simulink model "fermentation"  (R2019b)
settings: Solver=FixedStepAuto  StartTime=0.0  StopTime=stopTime  FixedStep=timeDelta  RelTol=1e-3
values from neighbouring files (symbols this model uses):
  a = 1000    [LoadDefaults.m]
  alpha0 = 70    [LoadDefaults.m]
  alpha1 = 0.143    [LoadDefaults.m]
  alpha2 = 4e-7    (= 4e-07)    [LoadDefaults.m]
  alpha3 = 1e-4    (= 0.0001)    [LoadDefaults.m]
  b = 0.6    [LoadDefaults.m]
  beta0 = 0.4    [LoadDefaults.m]
  Cab = Ca    (= 3)    [LoadDefaults.m]
  CL_init = GenRandomWithinRange ( CL_optimal)    [GenerateHistoricalBatches.m]    (also in LoadDefaults.m = 1.16)
  CLsat = 1.16    [LoadDefaults.m]
  CO2_init = 0.5    [LoadDefaults.m]
  Ed = 50000    [LoadDefaults.m]
  Eg = 5100    [LoadDefaults.m]
  F_init = 0    [LoadDefaults.m]
  Fa_init = 0    [LoadDefaults.m]
  Fa_max = 0.01/1000    (= 1e-05)    [LoadDefaults.m]
  Fb_init = 0    [LoadDefaults.m]
  Fb_max = 100/1000    (= 0.1)    [LoadDefaults.m]
  Fc_init = 0    [LoadDefaults.m]
  gamma0 = 1e-5    (= 1e-05)    [LoadDefaults.m]
  H_init = 10^(-pH_init)    [GenerateHistoricalBatches.m]    (also in LoadDefaults.m = 1e-05)
  K = 0.04    [LoadDefaults.m]
  K1 = 1e-10    [LoadDefaults.m]
  K2 = 7e-5    (= 7e-05)    [LoadDefaults.m]
  Kc_acid = 1e-4    (= 0.0001)    [LoadDefaults.m]
  Kc_base = 8e-4    (= 0.0008)    [LoadDefaults.m]
  Kc_cooling = 7    [LoadDefaults.m]
  kd = 1e33    (= 1e+33)    [LoadDefaults.m]
  kg = 7e3    (= 7000)    [LoadDefaults.m]
  KI = 0.1    [LoadDefaults.m]
  Kop = Kop_lim    (= 0.0005)    [LoadDefaults.m]
  Kox = Kox_lim    (= 0.02)    [LoadDefaults.m]
  Kp = 0.0002    [LoadDefaults.m]
  Kx = 0.15    [LoadDefaults.m]
  lambda0 = 1.0039e-4    (= 0.00010039)    [LoadDefaults.m]
  mo = 0.467    [LoadDefaults.m]
  mu_p = 0.005    [LoadDefaults.m]
  mu_x = 0.092    [LoadDefaults.m]
  mx = 0.014    [LoadDefaults.m]
  p = 3    [LoadDefaults.m]
  P_init = 0    [LoadDefaults.m]
  P_threshold = 1.3    [LoadDefaults.m]
  pH_init = GenRandomWithinRange ( pH_optimal )    [GenerateHistoricalBatches.m]    (also in LoadDefaults.m = -log10(H_init))
  q = 0    [LoadDefaults.m]
  Qrxn_init = 0    [LoadDefaults.m]
  R = 1.987    [LoadDefaults.m]
  rhoCp = 1500    [LoadDefaults.m]
  rq2 = 1.6783e-4    (= 0.00016783)    [LoadDefaults.m]
  S_init = GenRandomWithinRange ( S_optimal )    [GenerateHistoricalBatches.m]
  S_threshold = GenRandomWithinRange ( S_threshold_range )    [GenerateHistoricalBatches.m]    (also in LoadDefaults.m = 0.3)
  setpoint_H = 10^(-1*setpoint_pH)    (= 1e-05)    [LoadDefaults.m]
  setpoint_pH = 5    [LoadDefaults.m]
  setpoint_temp = 298    [LoadDefaults.m]
  setpointGap_pH = 0.01    [LoadDefaults.m]
  sf = 600    [LoadDefaults.m]
  T0 = 273    [LoadDefaults.m]
  T_init = 298    [LoadDefaults.m]
  tauD_acid = 0.125    [LoadDefaults.m]
  tauD_base = 0.2625    [LoadDefaults.m]
  tauD_cooling = 1.6    [LoadDefaults.m]
  tauI_acid = 8.4    [LoadDefaults.m]
  tauI_base = 4.2    [LoadDefaults.m]
  tauI_cooling = 0.5    [LoadDefaults.m]
  Tc = 273+16.8    (= 289.8)    [LoadDefaults.m]
  Th = 273+50    (= 323)    [LoadDefaults.m]
  timeDelta = 0.01    [LoadDefaults.m]
  Tv = 373    [LoadDefaults.m]
  V_init = GenRandomWithinRange ( V_optimal )    [GenerateHistoricalBatches.m]    (also in LoadDefaults.m = 100)
  X_init = GenRandomWithinRange ( X_range )    [GenerateHistoricalBatches.m]    (also in LoadDefaults.m = 0.1)
  Ypo = 0.20    (= 0.2)    [LoadDefaults.m]
  Yps = 0.90    (= 0.9)    [LoadDefaults.m]
  Yxo = 0.04    [LoadDefaults.m]
  Yxs = 0.45    [LoadDefaults.m]
undefined symbols (not defined in the file or in its folder): G_O2_mean, G_O2_std, rho_cCp_c, rq1
settings Model: Creator=Jedd  LastModifiedBy=jorsmond
settings DebuggingCC: SignalInfNanChecking=error

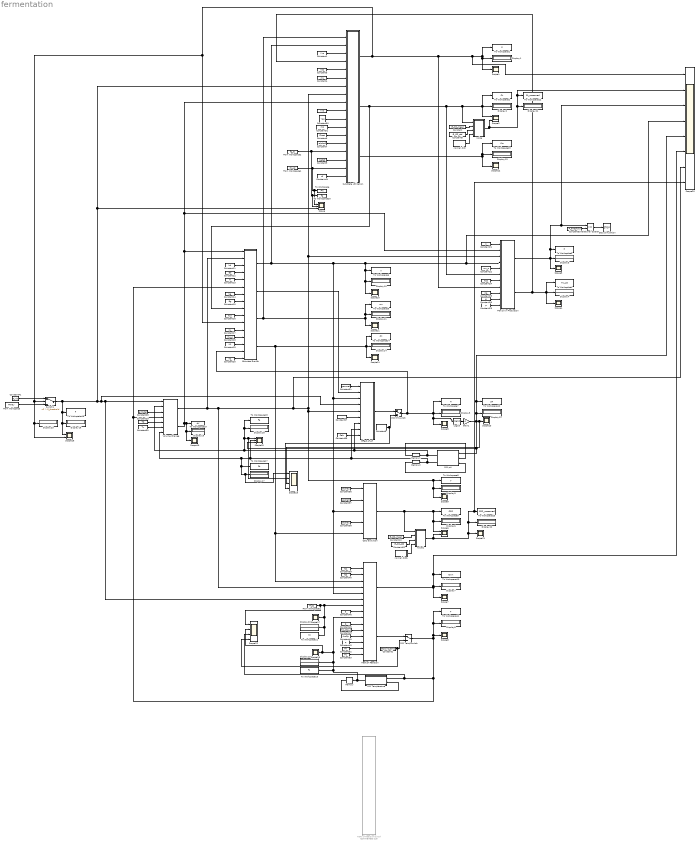
== system fermentation ==
  " " : Constant  Value=Yxo
  Biomass Growth : Subsystem
  CO2 evolution : Subsystem
  Constant : Constant  Value=G_O2_mean
  Constant1 : Constant  Value=Yxs
  Constant10 : Constant  Value=G_O2_mean
  Constant11 : Constant  Value=kd
  Constant12 : Constant  Value=Ed
  Constant13 : Constant  Value=R
  Constant14 : Constant  Value=kg
  Constant15 : Constant  Value=Eg
  Constant16 : Constant  Value=Kox
  Constant17 : Constant  Value=Kx
  Constant18 : Constant  Value=mu_x
  Constant19 : Constant  Value=K1
  Constant2 : Constant  Value=setpoint_temp
  Constant20 : Constant  Value=K2
  Constant21 : Constant  Value=K
  Constant22 : Constant  Value=mu_p
  Constant23 : Constant  Value=p
  Constant24 : Constant  Value=Kop
  Constant25 : Constant  Value=Kp
  Constant26 : Constant  Value=KI
  Constant27 : Constant  Value=timeDelta
  Constant28 : Constant  Value=lambda0
  Constant29 : Constant  Value=T0
  Constant3 : Constant  Value=Yps
  Constant30 : Constant  Value=Tv
  Constant31 : Constant  Value=gamma0
  Constant32 : Constant  Value=G_O2_std
  Constant33 : Constant  Value=P_threshold
  Constant35 : Constant  Value=Cab
  Constant36 : Constant  Value=alpha2
  Constant37 : Constant  Value=alpha3
  Constant38 : Constant  Value=alpha1
  Constant39 : Constant  Value=rq1
  Constant4 : Constant  Value=mx
  Constant40 : Constant  Value=rq2
  Constant41 : Constant  Value=F_init
  Constant43 : Constant  Value=q
  Constant44 : Constant  Value=sf
  Constant45 : Constant  Value=rhoCp
  Constant46 : Constant  Value=a
  Constant48 : Constant  Value=b
  Constant49 : Constant  Value=rho_cCp_c
  Constant5 : Constant  Value=setpoint_H
  Constant50 : Constant  Value=Ypo
  Constant51 : Constant  Value=mo
  Constant52 : Constant  Value=Th
  Constant53 : Constant  Value=Tc
  Constant6 : Constant  Value=CLsat
  Constant7 : Constant  Value=alpha0
  Constant8 : Constant  Value=G_O2_std
  Constant9 : Constant  Value=beta0
  Display{1..23} (23 alike) : Display
  Effect of pH : Subsystem
  From Workspace : FromWorkspace  VariableName=FArray  SampleTime=0
  From Workspace1 : FromWorkspace  VariableName=Pw_ts  SampleTime=timeDelta
  From Workspace2 : FromWorkspace  VariableName=fg_ts  SampleTime=timeDelta
  From Workspace3 : FromWorkspace  VariableName=Tf_ts  SampleTime=timeDelta
  Gain1 : Gain  Gain=-1
  Heat of Reaction : Subsystem
  Heat of Reaction(Cinar) : Subsystem  Commented=on
  Log10 : Math  Operator=log10  SignedPower=off  SaturateOnIntegerOverflow=on
  Memory : Memory  InitialCondition=Fc_init
  Memory1 : Memory  InitialCondition=Fa_init
  Memory2 : Memory  InitialCondition=Fb_init
  PID Temp switch : ManualSwitch
  PID Temperature : Subsystem
  PID [H] switch : ManualSwitch
  PID pH : Subsystem
  Penicillin Production : Subsystem
  Relational Operator : RelationalOperator  OutDataTypeStr=boolean  RndMeth=Simplest
  Scope : Scope  NumInputPorts=3
  Scope{1,3..5,7..15,17,19,21} (16 alike) : Scope
  Scope16 : Scope  NumInputPorts=2
  Scope18 : Scope  NumInputPorts=3
  Scope2 : Scope  NumInputPorts=2
  Scope20 : Scope  NumInputPorts=8
  Scope22 : Scope  NumInputPorts=4
  Scope23 : Scope  NumInputPorts=4
  Scope6 : Scope  NumInputPorts=2
  Stop Simulation : Stop
  Substrate Utilization : Subsystem
  Switch1 : Switch  Criteria=u2 > Threshold  Threshold=S_threshold
  To Workspace : ToWorkspace  VariableName=Pw  SaveFormat=Timeseries  SampleTime=-1
  To Workspace1 : ToWorkspace  VariableName=S  SaveFormat=Timeseries  SampleTime=-1
  To Workspace10 : ToWorkspace  VariableName=Qrxn  SaveFormat=Timeseries  SampleTime=-1
  To Workspace11 : ToWorkspace  VariableName=T  SaveFormat=Timeseries  SampleTime=-1
  To Workspace12 : ToWorkspace  VariableName=pH  SaveFormat=Timeseries  SampleTime=-1
  To Workspace13 : ToWorkspace  VariableName=Kla  SaveFormat=Timeseries  SampleTime=-1
  To Workspace14 : ToWorkspace  VariableName=dX  SaveFormat=Timeseries  SampleTime=-1
  To Workspace15 : ToWorkspace  VariableName=Fc  SaveFormat=Timeseries  SampleTime=-1
  To Workspace16 : ToWorkspace  VariableName=F  SaveFormat=Timeseries  SampleTime=-1
  To Workspace17 : ToWorkspace  VariableName=Fb  SaveFormat=Timeseries  SampleTime=-1
  To Workspace18 : ToWorkspace  VariableName=Fa  SaveFormat=Timeseries  SampleTime=-1
  To Workspace19 : ToWorkspace  VariableName=dV  SaveFormat=Timeseries  SampleTime=-1
  To Workspace2 : ToWorkspace  VariableName=CL  SaveFormat=Timeseries  SampleTime=-1
  To Workspace20 : ToWorkspace  VariableName=fg  SaveFormat=Timeseries  SampleTime=-1
  To Workspace21 : ToWorkspace  VariableName=Tf  SaveFormat=Timeseries  SampleTime=-1
  To Workspace22 : ToWorkspace  VariableName=CL_measured  SaveFormat=Timeseries  SampleTime=-1
  To Workspace23 : ToWorkspace  VariableName=CO2_measured  SaveFormat=Timeseries  SampleTime=-1
  To Workspace3 : ToWorkspace  VariableName=P  SaveFormat=Timeseries  SampleTime=-1
  To Workspace4 : ToWorkspace  VariableName=mu_pp  SaveFormat=Timeseries  SampleTime=-1
  To Workspace5 : ToWorkspace  VariableName=mu  SaveFormat=Timeseries  SampleTime=-1
  To Workspace6 : ToWorkspace  VariableName=X  SaveFormat=Timeseries  SampleTime=-1
  To Workspace7 : ToWorkspace  VariableName=H  SaveFormat=Timeseries  SampleTime=-1
  To Workspace8 : ToWorkspace  VariableName=V  SaveFormat=Timeseries  SampleTime=-1
  To Workspace9 : ToWorkspace  VariableName=CO2  SaveFormat=Timeseries  SampleTime=-1
  Volume Change : Subsystem
  noise : MATLAB Function  TreatAsAtomicUnit=on
  noise1 : MATLAB Function  TreatAsAtomicUnit=on
  normal dist : MATLAB Function  TreatAsAtomicUnit=on
  normal dist1 : MATLAB Function  TreatAsAtomicUnit=on
  wires:
  Biomass Growth/2(mu*X) -> Effect of pH/2(mu*X)
  Biomass Growth/4(dX/dt) -> Heat of Reaction/3(dX/dt), CO2 evolution/5(dX/dt), To Workspace14/1, Scope14/1, Display14/1
  Volume Change/2(dV/dt) -> Scope19/1, Display19/1, To Workspace19/1, Biomass Growth/1(dV/dt), Penicillin Production/2(dV/dt), Substrate Utilization/9(dV/dt)
  Constant1/1 -> Substrate Utilization/3(Yxs)
  Penicillin Production/2(mu_pp) -> Substrate Utilization/4(mu_pp), To Workspace4/1, Scope4/1, Display4/1
  Constant3/1 -> Substrate Utilization/5(Yps)
  Constant4/1 -> Substrate Utilization/6(mx)
  " "/1 -> Substrate Utilization/10(Yxo)
  Constant50/1 -> Substrate Utilization/11(Ypo)
  Constant51/1 -> Substrate Utilization/12(mo)
  Constant6/1 -> Substrate Utilization/13(CLsat)
  Constant7/1 -> Substrate Utilization/14(alpha0)
  From Workspace2/1 -> Scope/2, To Workspace20/1, Substrate Utilization/15(fg)
  Constant9/1 -> Substrate Utilization/16(beta0)
  From Workspace1/1 -> Scope/1, To Workspace/1, Substrate Utilization/17(Pw)
  Constant11/1 -> Biomass Growth/3(kd)
  Constant12/1 -> Biomass Growth/4(Ed)
  Constant13/1 -> Biomass Growth/5(R)
  Constant14/1 -> Biomass Growth/7(kg)
  Constant15/1 -> Biomass Growth/8(Eg)
  Constant16/1 -> Biomass Growth/10(Kox)
  Constant17/1 -> Biomass Growth/12(Kx)
  Constant18/1 -> Biomass Growth/13(mu_x)
  Constant19/1 -> Biomass Growth/14(K1)
  Constant20/1 -> Biomass Growth/16(K2)
  Constant21/1 -> Penicillin Production/1(K)
  Constant22/1 -> Penicillin Production/5(mu_p)
  Constant24/1 -> Penicillin Production/7(Kop)
  Constant25/1 -> Penicillin Production/9(Kp)
  Constant26/1 -> Penicillin Production/10(KI)
  Switch1/1 -> Scope16/1, Display16/1, To Workspace16/1, Substrate Utilization/7(F), Scope/3, Effect of pH/4(F), Heat of Reaction/6(F), Volume Change/1(F)  "F"
  Constant28/1 -> Volume Change/3(lambda0)
  Constant29/1 -> Volume Change/5(T0)
  Constant31/1 -> Effect of pH/1(gamma)
  Constant35/1 -> Effect of pH/9(Cab)
  Constant36/1 -> CO2 evolution/1(alpha2)
  Constant37/1 -> CO2 evolution/2(alpha3)
  Constant38/1 -> CO2 evolution/4(alpha1)
  Constant39/1 -> Heat of Reaction/1(rq1)
  Constant40/1 -> Heat of Reaction/2(rq2)
  From Workspace3/1 -> Scope22/1, To Workspace21/1, Display20/1, Scope17/1, Heat of Reaction/7(Tf)  "substrate feed temp"
  Constant45/1 -> Heat of Reaction/12(rhoCp)
  Constant46/1 -> Heat of Reaction/8(a)
  Constant48/1 -> Heat of Reaction/10(b)
  PID Temp switch/1 -> Biomass Growth/6(T), Volume Change/4(T), Scope22/3, PID Temperature/1(T), To Workspace11/1, Display8/1, Scope8/1  "T"
  Biomass Growth/1(X) -> Scope20/4, Penicillin Production/4(X), Scope10/1, Display10/1, To Workspace6/1, CO2 evolution/3(X), Heat of Reaction/5(X), Effect of pH/3(X), Substrate Utilization/2(X)  "biomass"
  Biomass Growth/3(mu) -> Substrate Utilization/1(mu), Scope11/1, To Workspace5/1, Display11/1
  Penicillin Production/1(P) -> Scope20/3, Relational Operator/1, To Workspace3/1, Scope3/1, Display3/1  "Penicillin"
  Constant49/1 -> Heat of Reaction/11(rho_cCp_c)
  Constant44/1 -> Substrate Utilization/18(sf)
  Heat of Reaction/2(T) -> PID Temp switch/1  "T"
  Constant2/1 -> Scope22/4, PID Temp switch/2
  Constant30/1 -> Volume Change/6(Tv)
  Effect of pH/1(H) -> PID [H] switch/1
  Constant5/1 -> Scope23/4, PID [H] switch/2  "SP"
  Constant23/1 -> Penicillin Production/11(p)
  Constant27/1 -> Effect of pH/6(timeDelta)
  Constant41/1 -> Switch1/1
  Substrate Utilization/1(S) -> Display23/1, Scope16/2, Switch1/2, Biomass Growth/11(S), Penicillin Production/8(S), Scope20/1, Scope1/1, Display1/1, To Workspace1/1  "Substrate"
  Constant43/1 -> Heat of Reaction/13(q)
  Constant52/1 -> Heat of Reaction/14(Th)
  Constant53/1 -> Heat of Reaction/15(Tc)
  PID [H] switch/1 -> Biomass Growth/15(H), Log10/1, Scope5/1, Display5/1, To Workspace7/1  "H"
  Log10/1 -> Gain1/1
  Volume Change/1(V) -> Heat of Reaction/4(V), Scope20/7, Effect of pH/5(V), Scope9/1, Display9/1, To Workspace8/1, Substrate Utilization/8(V), Penicillin Production/3(V), Biomass Growth/2(V)  "V"
  Substrate Utilization/3(Kla) -> Display13/1, To Workspace13/1, Scope12/1
  Heat of Reaction/1(Qrxn) -> Display7/1, Scope20/6, To Workspace10/1, Scope7/1  "Qrxn"
  Gain1/1 -> PID pH/1(PH), Scope18/3, Scope23/3, Scope13/1, Scope20/5, To Workspace12/1, Display12/1  "pH"
  Memory/1 -> PID Temperature/2(Fc,old)  "Fc(n-1)"
  PID Temperature/1(Fc,new) -> To Workspace15/1, Display15/1, Scope22/2, Scope15/1, Heat of Reaction/9(Fch), Memory/1  "Fc(n)"
  Memory1/1 -> PID pH/2(Fa,old)  "Fa(n-1)"
  Memory2/1 -> PID pH/3(Fb,old)  "Fb(n-1)"
  PID pH/1(Fa,new) -> To Workspace18/1, Display18/1, Scope23/2, Scope18/1, Volume Change/2(Fa), Effect of pH/7(Fa), Memory1/1  "Fa(n)"
  PID pH/2(Fb,new) -> Scope18/2, Scope23/1, Display17/1, To Workspace17/1, Volume Change/7(Fb), Effect of pH/8(Fb), Memory2/1  "Fb(n)"
  noise/1(y) -> Scope2/2, Display21/1, Scope20/2, To Workspace22/1  "Dissolved Oxygen"
  Substrate Utilization/2(CL) -> Biomass Growth/9(CL), Penicillin Production/6(CL), noise/1(u), Scope2/1, To Workspace2/1, Display2/1
  Constant/1 -> noise/2(mean)
  Constant8/1 -> noise/3(std)
  normal dist/1(y) -> noise/4(r)
  Constant32/1 -> noise1/3(std)
  Constant10/1 -> noise1/2(mean)
  normal dist1/1(y) -> noise1/4(r)
  CO2 evolution/1(CO2) -> noise1/1(u), Scope6/1, Display6/1, To Workspace9/1
  noise1/1(y) -> Scope6/2, Scope20/8, To Workspace23/1, Display22/1, Scope21/1  "CO2"
  Constant33/1 -> Relational Operator/2
  Relational Operator/1 -> Stop Simulation/1
  From Workspace/1 -> Switch1/3

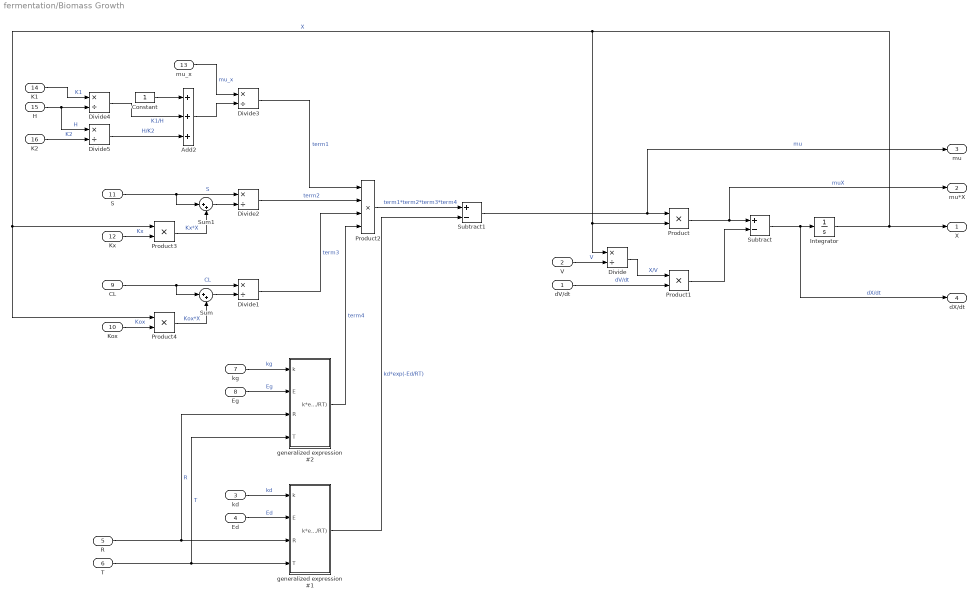
== system fermentation/Biomass Growth ==
  dV/dt : Inport
  V : Inport  Port=2
  kd : Inport  Port=3
  Ed : Inport  Port=4
  R : Inport  Port=5
  T : Inport  Port=6
  kg : Inport  Port=7
  Eg : Inport  Port=8
  CL : Inport  Port=9
  Kox : Inport  Port=10
  S : Inport  Port=11
  Kx : Inport  Port=12
  mu_x : Inport  Port=13
  K1 : Inport  Port=14
  H : Inport  Port=15
  K2 : Inport  Port=16
  Add2 : Sum  Inputs=3
  Constant : Constant
  Divide{,1..5} (6 alike) : Product  Inputs=*/
  Integrator : Integrator  InitialCondition=X_init
  Product{,1,3..4} (4 alike) : Product
  Product2 : Product  Inputs=4
  Subtract : Sum  Inputs=+-
  Subtract1 : Sum  Inputs=+-
  Sum : Sum  Inputs=|++
  Sum1 : Sum  Inputs=|++
  generalized expression #1 : Subsystem
  generalized expression #2 : Subsystem
  X : Outport
  mu*X : Outport  Port=2
  mu : Outport  Port=3
  dX/dt : Outport  Port=4
  wires:
  Product2/1 -> Subtract1/1  "term1*term2*term3*term4"
  Product/1 -> mu*X/1, Subtract/1  "muX"
  Divide/1 -> Product1/1  "X/V"
  Subtract/1 -> dX/dt/1, Integrator/1  "dX/dt"
  dV/dt/1 -> Product1/2  "dV/dt"
  V/1 -> Divide/2  "V"
  Product1/1 -> Subtract/2
  kd/1 -> generalized expression #1/1(k)  "kd"
  Ed/1 -> generalized expression #1/2(E)  "Ed"
  generalized expression #1/1(k*exp(-E/RT)) -> Subtract1/2  "kd*exp(-Ed/RT)"
  generalized expression #2/1(k*exp(-E/RT)) -> Product2/4  "term4"
  kg/1 -> generalized expression #2/1(k)  "kg"
  Eg/1 -> generalized expression #2/2(E)  "Eg"
  T/1 -> generalized expression #2/4(T), generalized expression #1/4(T)  "T"
  R/1 -> generalized expression #2/3(R), generalized expression #1/3(R)  "R"
  Subtract1/1 -> mu/1, Product/1  "mu"
  Divide1/1 -> Product2/3  "term3"
  CL/1 -> Sum/1, Divide1/1  "CL"
  Sum/1 -> Divide1/2
  Product4/1 -> Sum/2  "Kox*X"
  Kox/1 -> Product4/2  "Kox"
  Integrator/1 -> Divide/1, Product/2, Product4/1, Product3/1, X/1  "X"
  Kx/1 -> Product3/2  "Kx"
  Product3/1 -> Sum1/2  "Kx*X"
  Sum1/1 -> Divide2/2
  S/1 -> Sum1/1, Divide2/1  "S"
  Divide2/1 -> Product2/2  "term2"
  Divide3/1 -> Product2/1  "term1"
  mu_x/1 -> Divide3/1  "mu_x"
  Add2/1 -> Divide3/2
  Constant/1 -> Add2/1
  Divide4/1 -> Add2/2  "K1/H"
  Divide5/1 -> Add2/3  "H/K2"
  K1/1 -> Divide4/1  "K1"
  H/1 -> Divide5/1, Divide4/2  "H"
  K2/1 -> Divide5/2  "K2"

== system fermentation/CO2 evolution ==
  alpha2 : Inport
  alpha3 : Inport  Port=2
  X : Inport  Port=3
  alpha1 : Inport  Port=4
  dX/dt : Inport  Port=5
  Integrator : Integrator  InitialCondition=CO2_init
  Product : Product
  Product1 : Product
  Sum : Sum  Inputs=+++
  To Workspace11 : ToWorkspace  VariableName=dCO2  SaveFormat=Timeseries  SampleTime=-1
  CO2 : Outport
  wires:
  Integrator/1 -> CO2/1
  Sum/1 -> To Workspace11/1, Integrator/1
  alpha3/1 -> Sum/1
  Product/1 -> Sum/2
  alpha2/1 -> Product/1
  X/1 -> Product/2
  alpha1/1 -> Product1/1
  dX/dt/1 -> Product1/2
  Product1/1 -> Sum/3

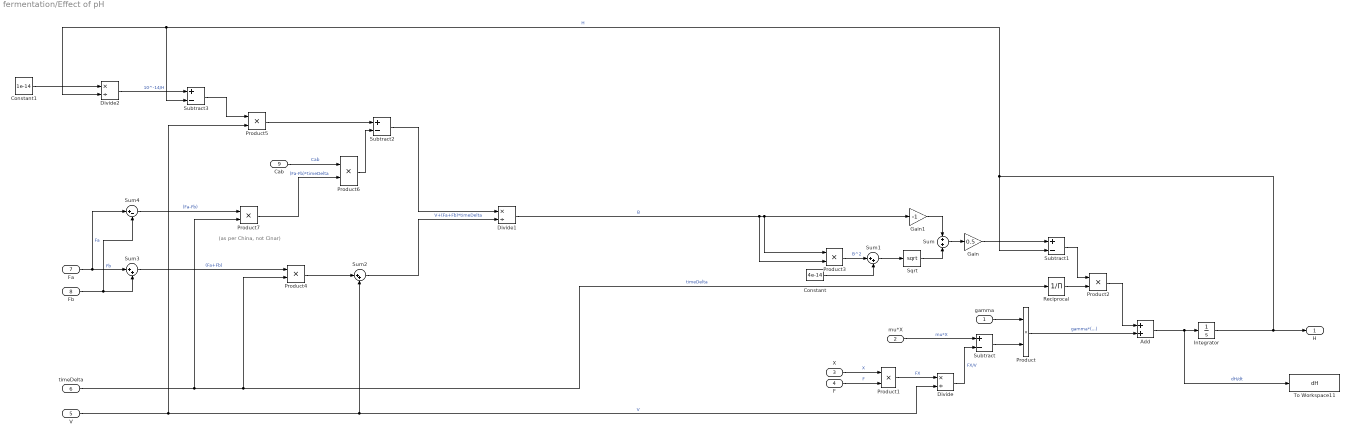
== system fermentation/Effect of pH ==
  note: (as per China, not Cinar)
  gamma : Inport
  mu*X : Inport  Port=2
  X : Inport  Port=3
  F : Inport  Port=4
  V : Inport  Port=5
  timeDelta : Inport  Port=6
  Fa : Inport  Port=7
  Fb : Inport  Port=8
  Cab : Inport  Port=9
  Add : Sum
  Constant : Constant  Value=4e-14
  Constant1 : Constant  Value=1e-14
  Divide : Product  Inputs=*/
  Divide1 : Product  Inputs=*/
  Divide2 : Product  Inputs=*/
  Gain : Gain  Gain=0.5
  Gain1 : Gain  Gain=-1
  Integrator : Integrator  InitialCondition=H_init
  Product{,1..7} (8 alike) : Product
  Reciprocal : Product  Inputs=/
  Sqrt : Sqrt  SaturateOnIntegerOverflow=on
  Subtract{,1..3} (4 alike) : Sum  Inputs=+-
  Sum : Sum
  Sum1 : Sum  Inputs=|++
  Sum2 : Sum  Inputs=|++
  Sum3 : Sum  Inputs=|++
  Sum4 : Sum  Inputs=|+-
  To Workspace11 : ToWorkspace  VariableName=dH  SaveFormat=Timeseries  SampleTime=-1
  H : Outport
  wires:
  Integrator/1 -> Subtract3/2, Divide2/2, Subtract1/2, H/1  "H"
  Product/1 -> Add/2  "gamma*(...)"
  gamma/1 -> Product/1
  Subtract/1 -> Product/2
  mu*X/1 -> Subtract/1  "mu*X"
  Divide/1 -> Subtract/2  "FX/V"
  X/1 -> Product1/1  "X"
  F/1 -> Product1/2  "F"
  Product1/1 -> Divide/1  "FX"
  V/1 -> Sum2/2, Divide/2, Product5/2  "V"
  Add/1 -> To Workspace11/1, Integrator/1  "dH/dt"
  Product2/1 -> Add/1
  Reciprocal/1 -> Product2/2
  timeDelta/1 -> Product7/2, Reciprocal/1, Product4/2  "timeDelta"
  Subtract1/1 -> Product2/1
  Gain/1 -> Subtract1/1
  Sum/1 -> Gain/1
  Gain1/1 -> Sum/1
  Divide1/1 -> Product3/2, Product3/1, Gain1/1  "B"
  Sqrt/1 -> Sum/2
  Sum1/1 -> Sqrt/1
  Constant/1 -> Sum1/2
  Product3/1 -> Sum1/1  "B^2"
  Sum2/1 -> Divide1/2  "V+(Fa+Fb)*timeDelta"
  Product4/1 -> Sum2/1
  Sum3/1 -> Product4/1  "(Fa+Fb)"
  Fb/1 -> Sum4/2, Sum3/2  "Fb"
  Subtract2/1 -> Divide1/1
  Product5/1 -> Subtract2/1
  Subtract3/1 -> Product5/1
  Divide2/1 -> Subtract3/1  "10^-14/H"
  Constant1/1 -> Divide2/1
  Product6/1 -> Subtract2/2
  Cab/1 -> Product6/1  "Cab"
  Fa/1 -> Sum4/1, Sum3/1  "Fa"
  Sum4/1 -> Product7/1  "(Fa-Fb)"
  Product7/1 -> Product6/2  "(Fa-Fb)*timeDelta"

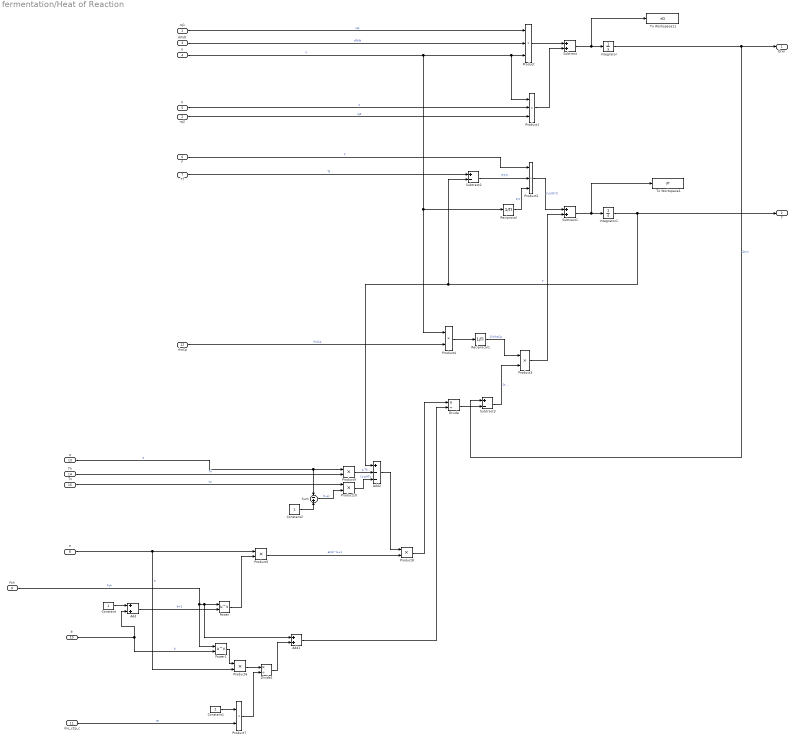
== system fermentation/Heat of Reaction ==
  rq1 : Inport
  rq2 : Inport  Port=2
  dX/dt : Inport  Port=3
  V : Inport  Port=4
  X : Inport  Port=5
  F : Inport  Port=6
  Tf : Inport  Port=7
  a : Inport  Port=8
  Fch : Inport  Port=9
  b : Inport  Port=10
  rho_cCp_c : Inport  Port=11
  rhoCp : Inport  Port=12
  q : Inport  Port=13
  Th : Inport  Port=14
  Tc : Inport  Port=15
  Add : Sum
  Add1 : Sum
  Add2 : Sum  Inputs=+--
  Constant : Constant
  Constant1 : Constant  Value=2
  Constant2 : Constant
  Divide : Product  Inputs=*/
  Divide1 : Product  Inputs=*/
  Integrator : Integrator  InitialCondition=Qrxn_init
  Integrator1 : Integrator  InitialCondition=T_init
  Power : Math  Operator=pow  SignedPower=off  SaturateOnIntegerOverflow=on
  Power1 : Math  Operator=pow  SignedPower=off  SaturateOnIntegerOverflow=on
  Product : Product  Inputs=3
  Product1 : Product  Inputs=3
  Product{3..10} (8 alike) : Product
  Product2 : Product  Inputs=3
  Reciprocal : Product  Inputs=/
  Reciprocal1 : Product  Inputs=/
  Subtract : Sum
  Subtract1 : Sum
  Subtract2 : Sum  Inputs=+-
  Subtract3 : Sum  Inputs=+-
  Sum : Sum  Inputs=-+
  To Workspace1 : ToWorkspace  VariableName=dT  SaveFormat=Timeseries  SampleTime=-1
  To Workspace11 : ToWorkspace  VariableName=dQ  SaveFormat=Timeseries  SampleTime=-1
  Qrxn : Outport
  T : Outport  Port=2
  wires:
  Integrator/1 -> Qrxn/1, Subtract3/1  "Qrxn"
  Subtract/1 -> To Workspace11/1, Integrator/1
  Product/1 -> Subtract/1
  rq1/1 -> Product/1  "rq1"
  dX/dt/1 -> Product/2  "dX/dt"
  Product1/1 -> Subtract/2
  rq2/1 -> Product1/3  "rq2"
  X/1 -> Product1/2  "X"
  Integrator1/1 -> Add2/1, Subtract2/2, T/1  "T"
  Subtract1/1 -> To Workspace1/1, Integrator1/1
  Product2/1 -> Subtract1/1  "F/V(Tf-T)"
  Subtract2/1 -> Product2/2  "(Tf-T)"
  F/1 -> Product2/1  "F"
  Tf/1 -> Subtract2/1  "Tf"
  Reciprocal/1 -> Product2/3  "1/V"
  V/1 -> Product1/1, Product/3, Reciprocal/1, Product4/1  "V"
  Product3/1 -> Subtract1/2
  Reciprocal1/1 -> Product3/1  "1/VrhoCp"
  Product4/1 -> Reciprocal1/1
  Subtract3/1 -> Product3/2  "Q-..."
  Divide/1 -> Subtract3/2
  Product5/1 -> Product8/2  "aFch^b+1"
  a/1 -> Product6/2, Product5/1  "a"
  Power/1 -> Product5/2
  Add/1 -> Power/2  "b+1"
  b/1 -> Power1/2, Add/2  "b"
  Constant/1 -> Add/1
  Add1/1 -> Divide/2
  Fch/1 -> Power1/1, Add1/1, Power/1  "Fch"
  Divide1/1 -> Add1/2
  Product6/1 -> Divide1/1
  Power1/1 -> Product6/1
  Product7/1 -> Divide1/2
  Constant1/1 -> Product7/1
  rho_cCp_c/1 -> Product7/2  "cp"
  rhoCp/1 -> Product4/2  "rhoCp"
  Product8/1 -> Divide/1
  Add2/1 -> Product8/1
  Product9/1 -> Add2/2  "q.Th"
  q/1 -> Sum/1, Product9/1  "q"
  Th/1 -> Product9/2  "Th"
  Product10/1 -> Add2/3  "(1-q)*Tc"
  Tc/1 -> Product10/1  "Tc"
  Sum/1 -> Product10/2  "(1-q)"
  Constant2/1 -> Sum/2

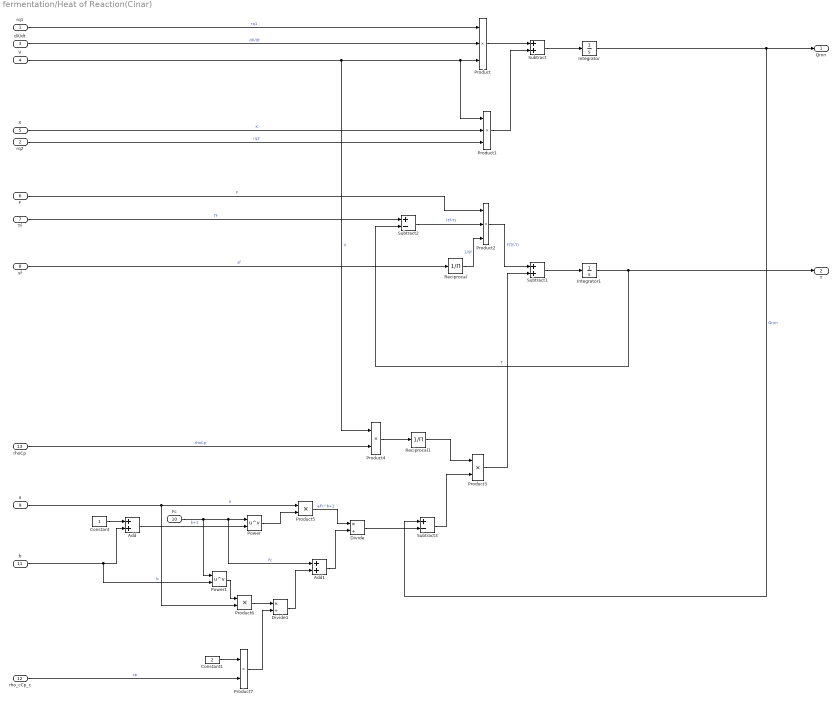
== system fermentation/Heat of Reaction(Cinar) ==
  rq1 : Inport
  rq2 : Inport  Port=2
  dX/dt : Inport  Port=3
  V : Inport  Port=4
  X : Inport  Port=5
  F : Inport  Port=6
  Tf : Inport  Port=7
  sf : Inport  Port=8
  a : Inport  Port=9
  Fc : Inport  Port=10
  b : Inport  Port=11
  rho_cCp_c : Inport  Port=12
  rhoCp : Inport  Port=13
  Add : Sum
  Add1 : Sum
  Constant : Constant
  Constant1 : Constant  Value=2
  Divide : Product  Inputs=*/
  Divide1 : Product  Inputs=*/
  Integrator : Integrator  InitialCondition=Qrxn_init
  Integrator1 : Integrator  InitialCondition=T_init
  Power : Math  Operator=pow  SignedPower=off  SaturateOnIntegerOverflow=on
  Power1 : Math  Operator=pow  SignedPower=off  SaturateOnIntegerOverflow=on
  Product : Product  Inputs=3
  Product1 : Product  Inputs=3
  Product2 : Product  Inputs=3
  Product{3..7} (5 alike) : Product
  Reciprocal : Product  Inputs=/
  Reciprocal1 : Product  Inputs=/
  Subtract : Sum
  Subtract1 : Sum
  Subtract2 : Sum  Inputs=+-
  Subtract3 : Sum  Inputs=+-
  Qrxn : Outport
  T : Outport  Port=2
  wires:
  Integrator/1 -> Qrxn/1, Subtract3/1  "Qrxn"
  Subtract/1 -> Integrator/1
  Product/1 -> Subtract/1
  rq1/1 -> Product/1  "rq1"
  dX/dt/1 -> Product/2  "dX/dt"
  V/1 -> Product1/1, Product/3, Product4/1  "V"
  Product1/1 -> Subtract/2
  rq2/1 -> Product1/3  "rq2"
  X/1 -> Product1/2  "X"
  Integrator1/1 -> Subtract2/2, T/1  "T"
  Subtract1/1 -> Integrator1/1
  Product2/1 -> Subtract1/1  "F(Tf-T)"
  Subtract2/1 -> Product2/2  "(Tf-T)"
  F/1 -> Product2/1  "F"
  Tf/1 -> Subtract2/1  "Tf"
  Reciprocal/1 -> Product2/3  "1/Sf"
  sf/1 -> Reciprocal/1  "sf"
  Product3/1 -> Subtract1/2
  Reciprocal1/1 -> Product3/1
  Product4/1 -> Reciprocal1/1
  Subtract3/1 -> Product3/2
  Divide/1 -> Subtract3/2
  Product5/1 -> Divide/1  "aFc^b+1"
  a/1 -> Product6/2, Product5/1  "a"
  Power/1 -> Product5/2
  Add/1 -> Power/2  "b+1"
  b/1 -> Power1/2, Add/2  "b"
  Constant/1 -> Add/1
  Add1/1 -> Divide/2
  Fc/1 -> Power1/1, Add1/1, Power/1  "Fc"
  Divide1/1 -> Add1/2
  Product6/1 -> Divide1/1
  Power1/1 -> Product6/1
  Product7/1 -> Divide1/2
  Constant1/1 -> Product7/1
  rho_cCp_c/1 -> Product7/2  "cp"
  rhoCp/1 -> Product4/2  "rhoCp"

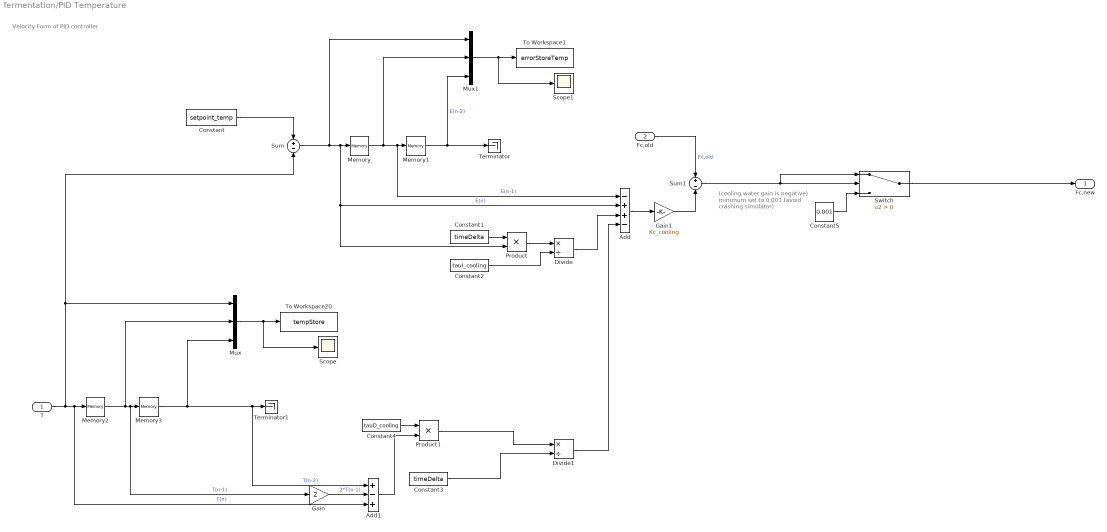
== system fermentation/PID Temperature ==
  note: Velocity Form of PID controller
  note: (cooling water gain is negative)
      | minimum set to 0.001
      | (avoid crashing simulator)
  T : Inport
  Fc,old : Inport  Port=2
  Add : Sum  Inputs=-++-
  Add1 : Sum  Inputs=+-+
  Constant : Constant  Value=setpoint_temp
  Constant1 : Constant  Value=timeDelta
  Constant2 : Constant  Value=tauI_cooling
  Constant3 : Constant  Value=timeDelta
  Constant4 : Constant  Value=tauD_cooling
  Constant5 : Constant  Value=0.001
  Divide : Product  Inputs=*/
  Divide1 : Product  Inputs=*/
  Gain : Gain  Gain=2
  Gain1 : Gain  Gain=Kc_cooling
  Memory : Memory
  Memory1 : Memory
  Memory2 : Memory  InitialCondition=T_init
  Memory3 : Memory  InitialCondition=T_init
  Mux : Mux  Inputs=3
  Mux1 : Mux  Inputs=3
  Product : Product
  Product1 : Product
  Scope : Scope
  Scope1 : Scope
  Sum : Sum  Inputs=+-
  Sum1 : Sum  Inputs=+-
  Switch : Switch  Criteria=u2 > Threshold
  Terminator : Terminator
  Terminator1 : Terminator
  To Workspace1 : ToWorkspace  VariableName=errorStoreTemp  SaveFormat=Timeseries  SampleTime=-1
  To Workspace20 : ToWorkspace  VariableName=tempStore  SaveFormat=Timeseries  SampleTime=-1
  Fc,new : Outport
  wires:
  Constant/1 -> Sum/1
  Sum/1 -> Mux1/1, Product/2, Add/2, Memory/1  "E(n)"
  Memory/1 -> Mux1/2, Add/1, Memory1/1  "E(n-1)"
  Memory1/1 -> Terminator/1, Mux1/3  "E(n-2)"
  T/1 -> Mux/1, Sum/2, Add1/3, Memory2/1  "T(n)"
  Memory2/1 -> Mux/2, Gain/1, Memory3/1  "T(n-1)"
  Memory3/1 -> Mux/3, Add1/1, Terminator1/1  "T(n-2)"
  Fc,old/1 -> Sum1/1  "Fc,old"
  Gain1/1 -> Sum1/2
  Add/1 -> Gain1/1
  Constant1/1 -> Product/1
  Product/1 -> Divide/1
  Divide/1 -> Add/3
  Constant2/1 -> Divide/2
  Divide1/1 -> Add/4
  Constant3/1 -> Divide1/2
  Product1/1 -> Divide1/1
  Constant4/1 -> Product1/1
  Add1/1 -> Product1/2
  Gain/1 -> Add1/2  "2*T(n-1)"
  Mux/1 -> Scope/1, To Workspace20/1
  Mux1/1 -> Scope1/1, To Workspace1/1
  Switch/1 -> Fc,new/1
  Sum1/1 -> Switch/1, Switch/2
  Constant5/1 -> Switch/3

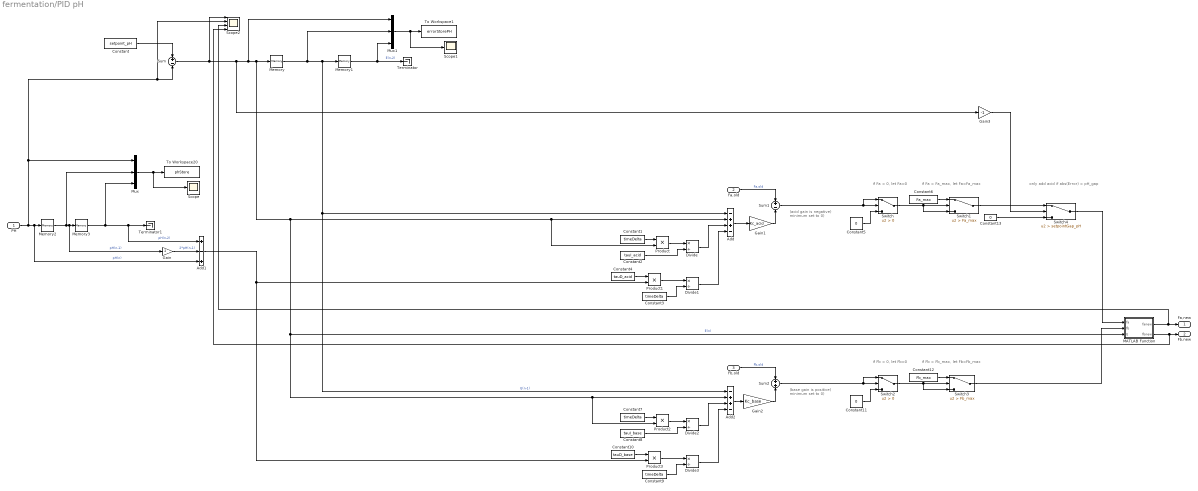
== system fermentation/PID pH ==
  note: (acid gain is negative)
      | minimum set to 0)
  note: if Fa < 0, let Fa=0
  note: if Fa > Fa_max, let Fa=Fa_max
  note: if Fb > Fb_max, let Fb=Fb_max
  note: if Fb < 0, let Fb=0
  note: (base gain is positive)
      | minimum set to 0)
  note: only add acid if abs(Error) > pH_gap
  PH : Inport
  Fa,old : Inport  Port=2
  Fb,old : Inport  Port=3
  Add : Sum  Inputs=-++-
  Add1 : Sum  Inputs=+-+
  Add2 : Sum  Inputs=-++-
  Constant : Constant  Value=setpoint_pH
  Constant{1,3,7,9} (4 alike) : Constant  Value=timeDelta
  Constant10 : Constant  Value=tauD_base
  Constant11 : Constant  Value=0
  Constant12 : Constant  Value=Fb_max
  Constant13 : Constant  Value=0
  Constant2 : Constant  Value=tauI_acid
  Constant4 : Constant  Value=tauD_acid
  Constant5 : Constant  Value=0
  Constant6 : Constant  Value=Fa_max
  Constant8 : Constant  Value=tauI_base
  Divide{,1..3} (4 alike) : Product  Inputs=*/
  Gain : Gain  Gain=2
  Gain1 : Gain  Gain=Kc_acid
  Gain2 : Gain  Gain=Kc_base
  Gain3 : Gain  Gain=-1
  MATLAB Function : MATLAB Function  TreatAsAtomicUnit=on
  Memory : Memory
  Memory1 : Memory
  Memory2 : Memory  InitialCondition=pH_init
  Memory3 : Memory  InitialCondition=pH_init
  Mux : Mux  Inputs=3
  Mux1 : Mux  Inputs=3
  Product{,1..3} (4 alike) : Product
  Scope : Scope
  Scope1 : Scope
  Scope2 : Scope  NumInputPorts=4
  Sum : Sum  Inputs=+-
  Sum1 : Sum  Inputs=+-
  Sum2 : Sum
  Switch : Switch  Criteria=u2 > Threshold
  Switch1 : Switch  Criteria=u2 > Threshold  Threshold=Fa_max
  Switch2 : Switch  Criteria=u2 > Threshold
  Switch3 : Switch  Criteria=u2 > Threshold  Threshold=Fb_max
  Switch4 : Switch  Criteria=u2 > Threshold  Threshold=setpointGap_pH
  Terminator : Terminator
  Terminator1 : Terminator
  To Workspace1 : ToWorkspace  VariableName=errorStorePH  SaveFormat=Timeseries  SampleTime=-1
  To Workspace20 : ToWorkspace  VariableName=phStore  SaveFormat=Timeseries  SampleTime=-1
  Fa,new : Outport
  Fb,new : Outport  Port=2
  wires:
  Constant/1 -> Sum/1
  Memory1/1 -> Terminator/1, Mux1/3  "E(n-2)"
  PH/1 -> Mux/1, Scope2/2, Sum/2, Add1/3, Memory2/1  "pH(n)"
  Memory2/1 -> Mux/2, Gain/1, Memory3/1  "pH(n-1)"
  Memory3/1 -> Mux/3, Add1/1, Terminator1/1  "pH(n-2)"
  Fa,old/1 -> Sum1/1  "Fa,old"
  Gain1/1 -> Sum1/2
  Add/1 -> Gain1/1
  Constant1/1 -> Product/1
  Product/1 -> Divide/1
  Divide/1 -> Add/3
  Constant2/1 -> Divide/2
  Divide1/1 -> Add/4
  Constant3/1 -> Divide1/2
  Product1/1 -> Divide1/1
  Constant4/1 -> Product1/1
  Gain/1 -> Add1/2  "2*pH(n-1)"
  Mux/1 -> Scope/1, To Workspace20/1
  Mux1/1 -> Scope1/1, To Workspace1/1
  Sum1/1 -> Switch/1, Switch/2
  Constant5/1 -> Switch/3
  Switch/1 -> Switch1/3, Switch1/2
  Constant6/1 -> Switch1/1
  Switch1/1 -> Switch4/1
  Sum2/1 -> Switch2/1, Switch2/2
  Constant10/1 -> Product3/1
  Add1/1 -> Product3/2, Product1/2
  Product3/1 -> Divide3/1
  Constant7/1 -> Product2/1
  Divide3/1 -> Add2/4
  Gain2/1 -> Sum2/2
  Divide2/1 -> Add2/3
  Add2/1 -> Gain2/1
  Constant8/1 -> Divide2/2
  Fb,old/1 -> Sum2/1  "Fb,old"
  Sum/1 -> Scope2/1, Gain3/1, Mux1/1, MATLAB Function/3(E), Product2/2, Add2/2, Product/2, Add/2, Memory/1  "E(n)"
  Constant9/1 -> Divide3/2
  Switch3/1 -> MATLAB Function/2(fb)
  Product2/1 -> Divide2/1
  Constant11/1 -> Switch2/3
  Switch2/1 -> Switch3/3, Switch3/2
  Constant12/1 -> Switch3/1
  Memory/1 -> Mux1/2, Add2/1, Add/1, Memory1/1  "E(n-1)"
  Switch4/1 -> MATLAB Function/1(fa)
  Constant13/1 -> Switch4/3
  MATLAB Function/1(fanew) -> Scope2/3, Fa,new/1
  MATLAB Function/2(fbnew) -> Scope2/4, Fb,new/1
  Gain3/1 -> Switch4/2

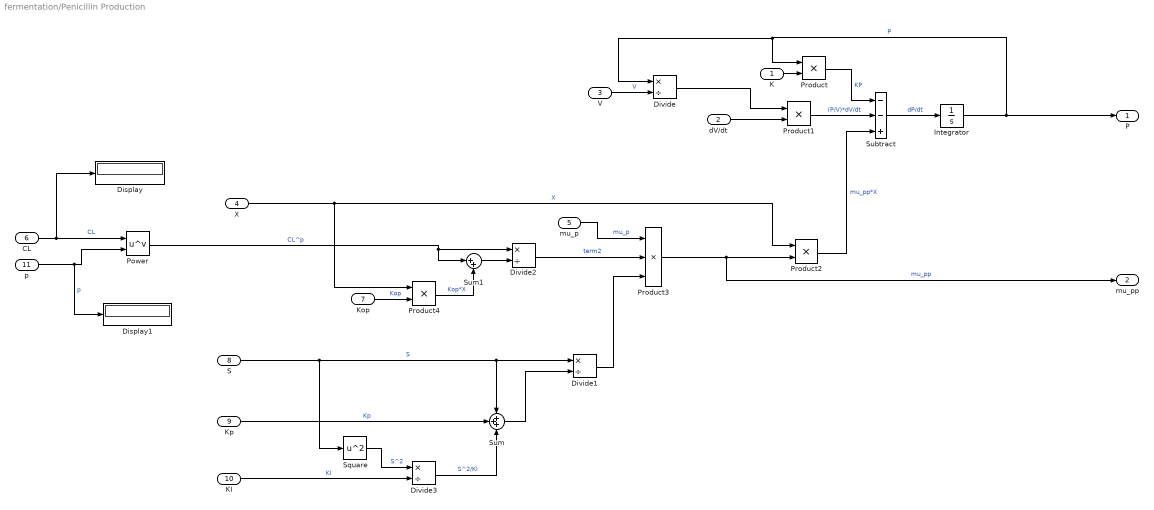
== system fermentation/Penicillin Production ==
  K : Inport
  dV/dt : Inport  Port=2
  V : Inport  Port=3
  X : Inport  Port=4
  mu_p : Inport  Port=5
  CL : Inport  Port=6
  Kop : Inport  Port=7
  S : Inport  Port=8
  Kp : Inport  Port=9
  KI : Inport  Port=10
  p : Inport  Port=11
  Display : Display
  Display1 : Display
  Divide{,1..3} (4 alike) : Product  Inputs=*/
  Integrator : Integrator  InitialCondition=P_init
  Power : Math  Operator=pow  SignedPower=off  SaturateOnIntegerOverflow=on
  Product{,1..2,4} (4 alike) : Product
  Product3 : Product  Inputs=3
  Square : Math  Operator=square  SignedPower=off  SaturateOnIntegerOverflow=on
  Subtract : Sum  Inputs=--+
  Sum : Sum  Inputs=+++
  Sum1 : Sum  Inputs=|++
  P : Outport
  mu_pp : Outport  Port=2
  wires:
  Integrator/1 -> Divide/1, Product/1, P/1  "P"
  Subtract/1 -> Integrator/1  "dP/dt"
  Product2/1 -> Subtract/3  "mu_pp*X"
  Product/1 -> Subtract/1  "KP"
  K/1 -> Product/2
  Product1/1 -> Subtract/2  "(P/V)*dV/dt"
  dV/dt/1 -> Product1/2
  Divide/1 -> Product1/1
  V/1 -> Divide/2  "V"
  Product3/1 -> mu_pp/1, Product2/2  "mu_pp"
  mu_p/1 -> Product3/1  "mu_p"
  Divide2/1 -> Product3/2  "term2"
  Product4/1 -> Sum1/2  "Kop*X"
  Kop/1 -> Product4/2  "Kop"
  Sum1/1 -> Divide2/2
  X/1 -> Product4/1, Product2/1  "X"
  Power/1 -> Sum1/1, Divide2/1  "CL^p"
  Divide1/1 -> Product3/3
  S/1 -> Square/1, Divide1/1, Sum/1  "S"
  Sum/1 -> Divide1/2
  Kp/1 -> Sum/2  "Kp"
  Divide3/1 -> Sum/3  "S^2/KI"
  Square/1 -> Divide3/1  "S^2"
  KI/1 -> Divide3/2  "KI"
  CL/1 -> Display/1, Power/1  "CL"
  p/1 -> Display1/1, Power/2  "p"

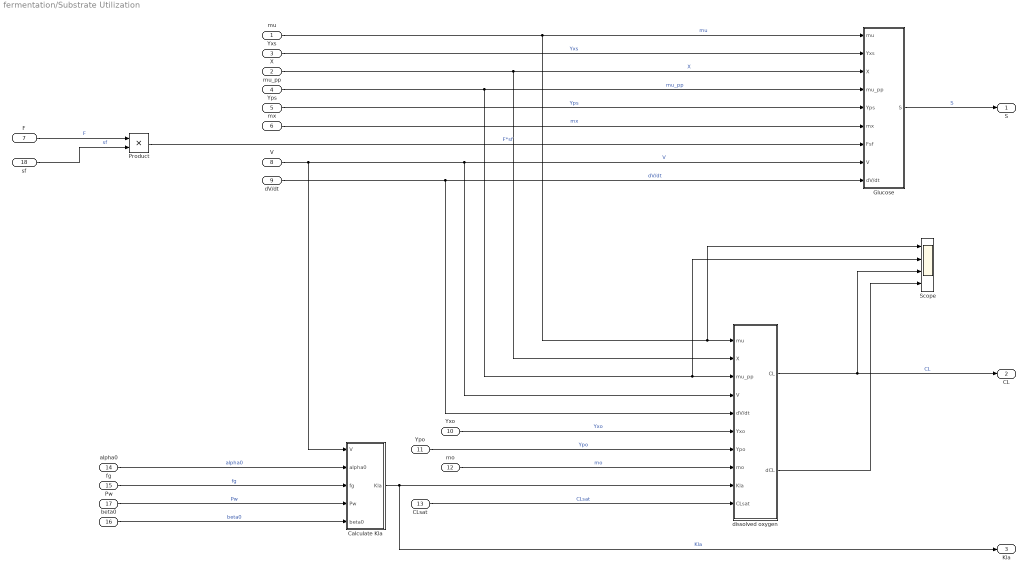
== system fermentation/Substrate Utilization ==
  mu : Inport
  X : Inport  Port=2
  Yxs : Inport  Port=3
  mu_pp : Inport  Port=4
  Yps : Inport  Port=5
  mx : Inport  Port=6
  F : Inport  Port=7
  V : Inport  Port=8
  dV/dt : Inport  Port=9
  Yxo : Inport  Port=10
  Ypo : Inport  Port=11
  mo : Inport  Port=12
  CLsat : Inport  Port=13
  alpha0 : Inport  Port=14
  fg : Inport  Port=15
  beta0 : Inport  Port=16
  Pw : Inport  Port=17
  sf : Inport  Port=18
  Calculate Kla : Subsystem
  Glucose : Subsystem
  Product : Product
  Scope : Scope  NumInputPorts=4
  dissolved oxygen : Subsystem
  S : Outport
  CL : Outport  Port=2
  Kla : Outport  Port=3
  wires:
  mu/1 -> Glucose/1(mu), Scope/1, dissolved oxygen/1(mu)  "mu"
  Yxs/1 -> Glucose/2(Yxs)  "Yxs"
  X/1 -> Glucose/3(X), dissolved oxygen/2(X)  "X"
  mu_pp/1 -> Glucose/4(mu_pp), Scope/2, dissolved oxygen/3(mu_pp)  "mu_pp"
  Yps/1 -> Glucose/5(Yps)  "Yps"
  mx/1 -> Glucose/6(mx)  "mx"
  Product/1 -> Glucose/7(Fsf)  "F*sf"
  V/1 -> dissolved oxygen/4(V), Glucose/8(V), Calculate Kla/1(V)  "V"
  dV/dt/1 -> Glucose/9(dV/dt), dissolved oxygen/5(dV/dt)  "dV/dt"
  Glucose/1(S) -> S/1  "S"
  Yxo/1 -> dissolved oxygen/6(Yxo)  "Yxo"
  Ypo/1 -> dissolved oxygen/7(Ypo)  "Ypo"
  mo/1 -> dissolved oxygen/8(mo)  "mo"
  CLsat/1 -> dissolved oxygen/10(CLsat)  "CLsat"
  dissolved oxygen/1(CL) -> CL/1, Scope/3  "CL"
  alpha0/1 -> Calculate Kla/2(alpha0)  "alpha0"
  fg/1 -> Calculate Kla/3(fg)  "fg"
  Pw/1 -> Calculate Kla/4(Pw)  "Pw"
  beta0/1 -> Calculate Kla/5(beta0)  "beta0"
  Calculate Kla/1(Kla) -> Kla/1, dissolved oxygen/9(Kla)  "Kla"
  F/1 -> Product/1  "F"
  sf/1 -> Product/2  "sf"
  dissolved oxygen/2(dCL) -> Scope/4

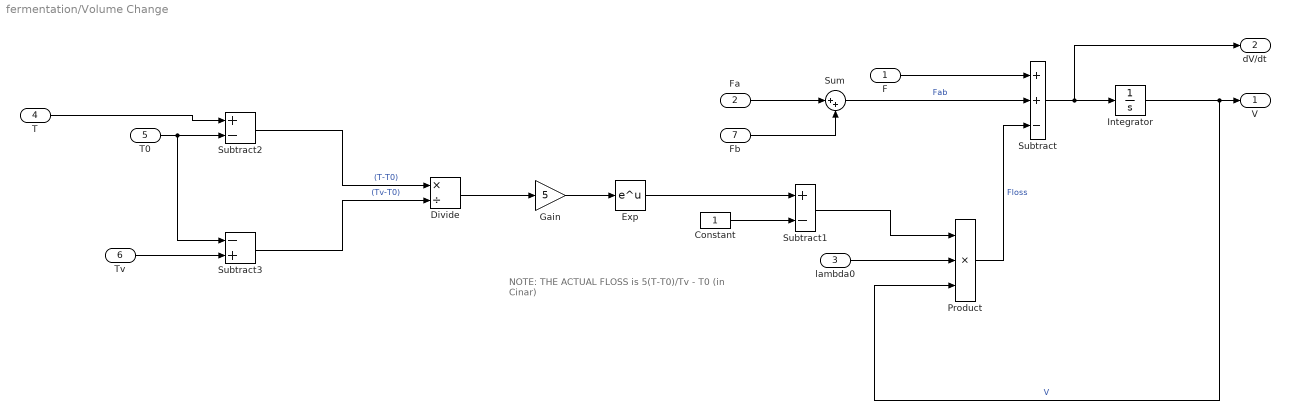
== system fermentation/Volume Change ==
  note: NOTE: THE ACTUAL FLOSS is 5(T-T0)/Tv - T0
      | (in Cinar)
  F : Inport
  Fa : Inport  Port=2
  lambda0 : Inport  Port=3
  T : Inport  Port=4
  T0 : Inport  Port=5
  Tv : Inport  Port=6
  Fb : Inport  Port=7
  Constant : Constant
  Divide : Product  Inputs=*/
  Exp : Math  SignedPower=off  SaturateOnIntegerOverflow=on
  Gain : Gain  Gain=5
  Integrator : Integrator  InitialCondition=V_init
  Product : Product  Inputs=3
  Subtract : Sum  Inputs=++-
  Subtract1 : Sum  Inputs=+-
  Subtract2 : Sum  Inputs=+-
  Subtract3 : Sum  Inputs=-+
  Sum : Sum  Inputs=|++
  V : Outport
  dV/dt : Outport  Port=2
  wires:
  Integrator/1 -> Product/3, V/1  "V"
  Subtract/1 -> dV/dt/1, Integrator/1
  Sum/1 -> Subtract/2  "Fab"
  F/1 -> Subtract/1
  Product/1 -> Subtract/3  "Floss"
  lambda0/1 -> Product/2
  Subtract1/1 -> Product/1
  Constant/1 -> Subtract1/2
  Exp/1 -> Subtract1/1
  Gain/1 -> Exp/1
  Divide/1 -> Gain/1
  T/1 -> Subtract2/1
  Subtract2/1 -> Divide/1  "(T-T0)"
  Subtract3/1 -> Divide/2  "(Tv-T0)"
  T0/1 -> Subtract3/1, Subtract2/2
  Tv/1 -> Subtract3/2
  Fb/1 -> Sum/2
  Fa/1 -> Sum/1

== system fermentation/Biomass Growth/generalized expression #1 ==
  k : Inport
  E : Inport  Port=2
  R : Inport  Port=3
  T : Inport  Port=4
  Constant : Constant  Value=-1
  Divide1 : Product  Inputs=*/
  Exp : Math  SignedPower=off  SaturateOnIntegerOverflow=on
  Product3 : Product
  Product4 : Product  Inputs=3
  k*exp(-E/RT) : Outport
  wires:
  T/1 -> Product4/2
  k/1 -> Product3/1  "k"
  Exp/1 -> Product3/2  "exp(..)"
  Product3/1 -> k*exp(-E/RT)/1
  Product4/1 -> Divide1/2  "-RT"
  E/1 -> Divide1/1  "E"
  Divide1/1 -> Exp/1  "-E/RT"
  Constant/1 -> Product4/3
  R/1 -> Product4/1

== system fermentation/Biomass Growth/generalized expression #2 ==
  k : Inport
  E : Inport  Port=2
  R : Inport  Port=3
  T : Inport  Port=4
  Constant : Constant  Value=-1
  Divide1 : Product  Inputs=*/
  Exp : Math  SignedPower=off  SaturateOnIntegerOverflow=on
  Product3 : Product
  Product4 : Product  Inputs=3
  k*exp(-E/RT) : Outport
  wires:
  T/1 -> Product4/2
  k/1 -> Product3/1  "k"
  Exp/1 -> Product3/2  "exp(..)"
  Product3/1 -> k*exp(-E/RT)/1
  Product4/1 -> Divide1/2  "-RT"
  E/1 -> Divide1/1  "E"
  Divide1/1 -> Exp/1  "-E/RT"
  Constant/1 -> Product4/3
  R/1 -> Product4/1

== system fermentation/Substrate Utilization/Calculate Kla ==
  V : Inport
  alpha0 : Inport  Port=2
  fg : Inport  Port=3
  Pw : Inport  Port=4
  beta0 : Inport  Port=5
  Divide2 : Product  Inputs=*/
  Power : Math  Operator=pow  SignedPower=off  SaturateOnIntegerOverflow=on
  Product6 : Product  Inputs=3
  Sqrt : Sqrt  SaturateOnIntegerOverflow=on
  Kla : Outport
  wires:
  Pw/1 -> Divide2/1
  Power/1 -> Product6/3
  Product6/1 -> Kla/1  "Kla"
  Sqrt/1 -> Product6/2  "sqrt(fg)"
  fg/1 -> Sqrt/1
  Divide2/1 -> Power/1
  alpha0/1 -> Product6/1
  V/1 -> Divide2/2
  beta0/1 -> Power/2

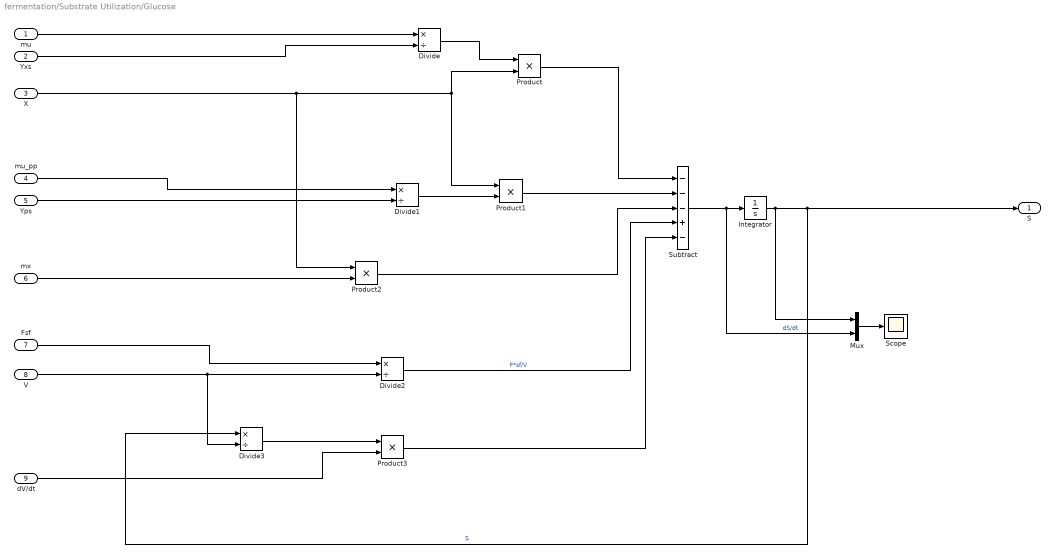
== system fermentation/Substrate Utilization/Glucose ==
  mu : Inport
  Yxs : Inport  Port=2
  X : Inport  Port=3
  mu_pp : Inport  Port=4
  Yps : Inport  Port=5
  mx : Inport  Port=6
  Fsf : Inport  Port=7
  V : Inport  Port=8
  dV/dt : Inport  Port=9
  Divide{,1..3} (4 alike) : Product  Inputs=*/
  Integrator : Integrator  InitialCondition=S_init
  Mux : Mux  Inputs=2
  Product{,1..3} (4 alike) : Product
  Scope : Scope
  Subtract : Sum  Inputs=---+-
  S : Outport
  wires:
  Integrator/1 -> Mux/1, S/1, Divide3/1  "S"
  Product2/1 -> Subtract/3
  Divide3/1 -> Product3/1
  Divide1/1 -> Product1/2
  Product1/1 -> Subtract/2
  V/1 -> Divide3/2, Divide2/2
  Divide/1 -> Product/1
  Divide2/1 -> Subtract/4  "F*sf/V"
  Subtract/1 -> Mux/2, Integrator/1  "dS/dt"
  X/1 -> Product2/1, Product1/1, Product/2
  Product3/1 -> Subtract/5
  mu/1 -> Divide/1
  Product/1 -> Subtract/1
  mx/1 -> Product2/2
  dV/dt/1 -> Product3/2
  Fsf/1 -> Divide2/1
  mu_pp/1 -> Divide1/1
  Yps/1 -> Divide1/2
  Yxs/1 -> Divide/2
  Mux/1 -> Scope/1

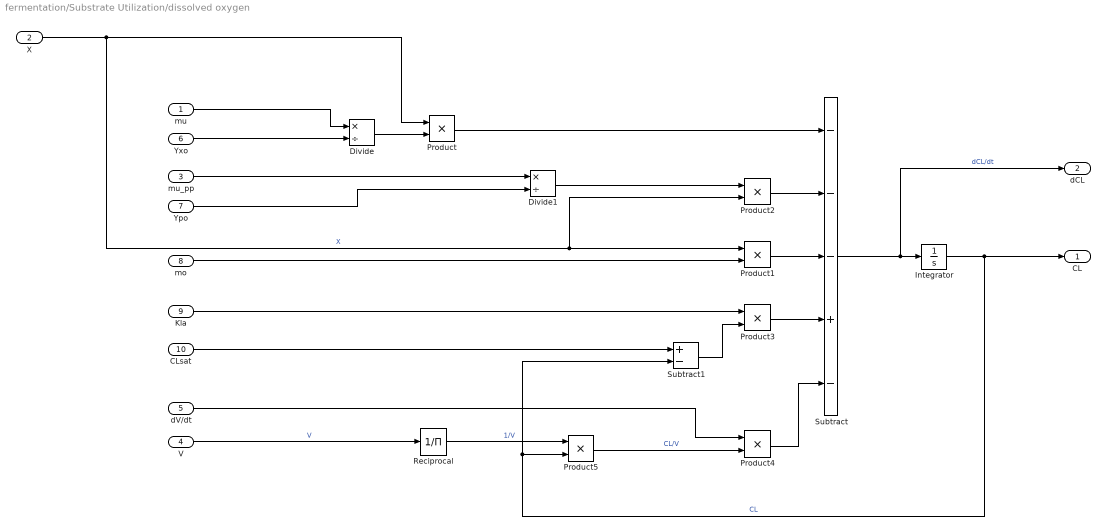
== system fermentation/Substrate Utilization/dissolved oxygen ==
  mu : Inport
  X : Inport  Port=2
  mu_pp : Inport  Port=3
  V : Inport  Port=4
  dV/dt : Inport  Port=5
  Yxo : Inport  Port=6
  Ypo : Inport  Port=7
  mo : Inport  Port=8
  Kla : Inport  Port=9
  CLsat : Inport  Port=10
  Divide : Product  Inputs=*/
  Divide1 : Product  Inputs=*/
  Integrator : Integrator  InitialCondition=CL_init
  Product{,1..5} (6 alike) : Product
  Reciprocal : Product  Inputs=/
  Subtract : Sum  Inputs=---+-
  Subtract1 : Sum  Inputs=+-
  CL : Outport
  dCL : Outport  Port=2
  wires:
  Product2/1 -> Subtract/2
  Product/1 -> Subtract/1
  Divide/1 -> Product/2
  X/1 -> Product/1, Product2/2, Product1/1  "X"
  Product3/1 -> Subtract/4
  Integrator/1 -> CL/1, Product5/2, Subtract1/2  "CL"
  Ypo/1 -> Divide1/2
  Divide1/1 -> Product2/1
  mo/1 -> Product1/2
  Subtract/1 -> dCL/1, Integrator/1  "dCL/dt"
  Subtract1/1 -> Product3/2
  mu_pp/1 -> Divide1/1
  Reciprocal/1 -> Product5/1  "1/V"
  Product5/1 -> Product4/2  "CL/V"
  Product1/1 -> Subtract/3
  Product4/1 -> Subtract/5
  Yxo/1 -> Divide/2
  mu/1 -> Divide/1
  CLsat/1 -> Subtract1/1
  V/1 -> Reciprocal/1  "V"
  dV/dt/1 -> Product4/1
  Kla/1 -> Product3/1

== matlab function fermentation/PID pH/MATLAB Function ==
  data: fa input; fanew output; fb input; fbnew output; E input
function [fanew,fbnew] = fcn(fa,fb, E)
% if fa >0 && fb > 0
%     disp('warning, acid and base feeding at the same time.');
%     if E > 0
%         disp('acid takes preference');
%         fanew = fa;
%         fbnew = 0;
%     else
%         disp('base takes preference');
%         fanew=0;
%         fbnew = fb;
%     end
% else
%     fanew=fa;
%     fbnew=fb;
% end
    
fanew = fa;
fbnew = fb;

== matlab function fermentation/noise ==
  data: u input; y output; mean input; std input; r input
function y = fcn(u, mean, std, r)

y = u + mean + std*r;

== matlab function fermentation/normal dist ==
  data: y output
function y = fcn()

y = randn(1,1);

== matlab function fermentation/noise1 ==
  data: u input; y output; mean input; std input; r input
function y = fcn(u, mean, std, r)

y = u + mean + std*r;

== matlab function fermentation/normal dist1 ==
  data: y output
function y = fcn()

y = randn(1,1);
